simulink model "preSAE"  (R2020a)
settings: Solver=VariableStepAuto  StartTime=0.0  StopTime=stoptime  RelTol=1e-3
values from neighbouring files (symbols this model uses):
  A = [Xu Xw -aa0*U0 -g*cos(tt0) ... (first row only)    [Model.m]
  B = [Xde Xdt ... (first row only)    [Model.m]
  C = eye(4)    [Model.m]
  D = zeros(4,2)    [Model.m]
  stoptime = 500    [Model.m]
settings Model: Creator=beapedroso  LastModifiedBy=tfesc
settings DataIOCC: ReturnWorkspaceOutputs=off
settings DebuggingCC: ArithmeticOperatorsInVariantConditions=warning
settings SFSimCC: SimUseLocalCustomCode=off  CustomCodeUndefinedFunction=UseInterfaceOnly
settings RTWCC: RTWUseLocalCustomCode=off

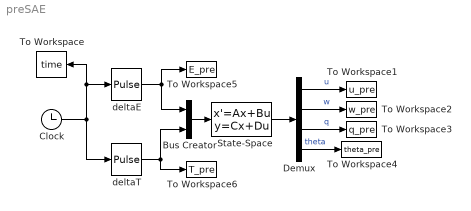
== system preSAE ==
  Bus Creator : BusCreator  Inputs=2
  Clock : Clock
  Demux : Demux
  State-Space : StateSpace  A=A  B=B  C=C  D=D  InitialCondition=0
  To Workspace : ToWorkspace  VariableName=time  SampleTime=-1
  To Workspace1 : ToWorkspace  VariableName=u_pre  SampleTime=-1
  To Workspace2 : ToWorkspace  VariableName=w_pre  SampleTime=-1
  To Workspace3 : ToWorkspace  VariableName=q_pre  SampleTime=-1
  To Workspace4 : ToWorkspace  VariableName=theta_pre  SampleTime=-1
  To Workspace5 : ToWorkspace  VariableName=E_pre  SampleTime=-1
  To Workspace6 : ToWorkspace  VariableName=T_pre  SampleTime=-1
  "deltaE " : DiscretePulseGenerator  PulseType=Time based  TimeSource=Use external signal  Amplitude=3*3.14/180  Period=stoptime  PulseWidth=15  PhaseDelay=300
  deltaT : DiscretePulseGenerator  PulseType=Time based  TimeSource=Use external signal  Amplitude=0.1  Period=stoptime  PulseWidth=10  PhaseDelay=50
  wires:
  Demux/2 -> To Workspace2/1  "w"
  Demux/4 -> To Workspace4/1  "theta"
  State-Space/1 -> Demux/1
  Demux/1 -> To Workspace1/1  "u"
  Demux/3 -> To Workspace3/1  "q"
  deltaT/1 -> Bus Creator/2, To Workspace6/1
  Bus Creator/1 -> State-Space/1
  "deltaE "/1 -> Bus Creator/1, To Workspace5/1
  Clock/1 -> deltaT/1, To Workspace/1, "deltaE "/1
